simulink model "heater_model"  (R2022b)
settings: Solver=FixedStepAuto  StartTime=0.0  StopTime=10.0  FixedStep=1/360  RelTol=1e-3
values from neighbouring files (symbols this model uses):
  c = 1005.4    [house_heat_data.mat]
  Mdot = 3600    [house_heat_data.mat]
  THeater = 50    [house_heat_data.mat]
settings Model: Creator=bneiswan  LastModifiedBy=bensweet
settings SolverCC: AlgebraicLoopSolver=TrustRegion
settings DataIOCC: ReturnWorkspaceOutputs=off
settings DebuggingCC: UnconnectedInputMsg=warning  UnconnectedOutputMsg=warning  UnconnectedLineMsg=warning  SFMachineParentedDataDiag=warning
settings ModelReferenceCC: EnableRefExpFcnMdlSchedulingChecks=on
settings RTWCC: DLArmComputeVersion=19.05

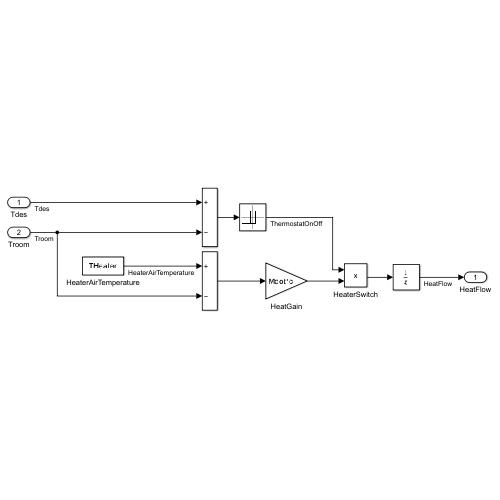
[thumbnail: Simulink's stored preview of the top-level diagram]
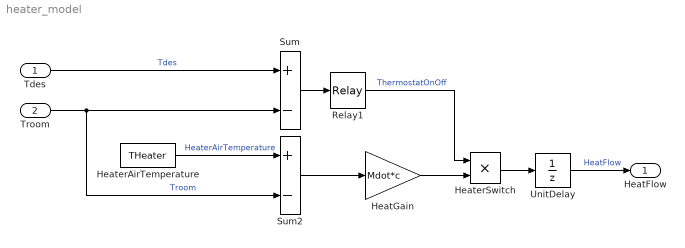
== system heater_model ==
  Tdes : Inport  PortDimensions=1  SampleTime=1/360
  Troom : Inport  Port=2  PortDimensions=1  SampleTime=1/360
  HeatGain : Gain  Gain=Mdot*c
  HeaterAirTemperature : Constant  Value=THeater
  HeaterSwitch : Product  RndMeth=Zero
  Relay1 : Relay  OnSwitchValue=1  OffSwitchValue=-1
  Sum : Sum  Inputs=+-  InputSameDT=on  SaturateOnIntegerOverflow=on  OutDataTypeStr=Inherit: Same as first input
  Sum2 : Sum  Inputs=+-
  UnitDelay : UnitDelay  SampleTime=1/360  HasFrameUpgradeWarning=on
  HeatFlow : Outport  PortDimensions=1  SampleTime=1/360  VectorParamsAs1DForOutWhenUnconnected=off
  wires:
  Sum/1 -> Relay1/1
  Relay1/1 -> HeaterSwitch/1  "ThermostatOnOff"
  HeaterSwitch/1 -> UnitDelay/1
  Troom/1 -> Sum/2, Sum2/2  "Troom"
  UnitDelay/1 -> HeatFlow/1  "HeatFlow"
  HeatGain/1 -> HeaterSwitch/2
  HeaterAirTemperature/1 -> Sum2/1  "HeaterAirTemperature"
  Sum2/1 -> HeatGain/1
  Tdes/1 -> Sum/1  "Tdes"
